simulink model "Synch_Gen1"  (Simulink 4.00)
settings: Solver=ode23tb  StartTime=0.0  StopTime=1
InitFcn:
  | powericon('psbinitsys',bdroot);
libraries: powerlib2 x8, powerlib_extras x3
settings Model: LastModifiedBy=ieao  SaveTime=off  SaveOutput=off  LimitDataPoints=off  BlockReductionOpt=off

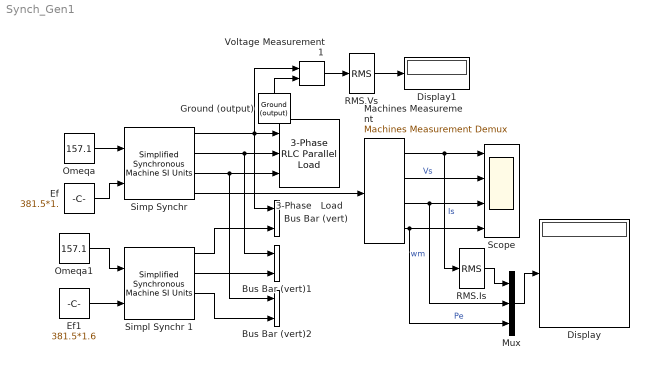
== system Synch_Gen1 ==
  3-Phase   Load : powerlib_extras/Three-Phase Library/3-Phase RLC Parallel Load  Vpp=380  fn=50  P3=100e3  QL3=50e3  QC3=0
  Bus Bar (vert) : powerlib2/Connectors/Bus Bar (vert)  Tag=PoWeRsYsTeMbLoCk  entrees=2  sorties=0  PSBOutputType=11111111111111111111111111111111111111111111111111111111111111111111111111111111111111111
  Bus Bar (vert)1 : powerlib2/Connectors/Bus Bar (vert)  Tag=PoWeRsYsTeMbLoCk  entrees=2  sorties=0  PSBOutputType=11111111111111111111111111111111111111111111111111111111111111111111111111111111111111111
  Bus Bar (vert)2 : powerlib2/Connectors/Bus Bar (vert)  Tag=PoWeRsYsTeMbLoCk  entrees=2  sorties=0  PSBOutputType=11111111111111111111111111111111111111111111111111111111111111111111111111111111111111111
  Display : Display
      settings: Format=short  SampleTime=0
  Display1 : Display
      settings: Format=short  SampleTime=0
  Ef : Constant  Value=381.5*1.
  Ef1 : Constant  Value=381.5*1.6
  Ground (output) : powerlib2/Connectors/Ground (output)  Tag=PoWeRsYsTeMbLoCk  Orientation=up  PSBOutputType=1
  Machines Measurement : powerlib2/Machines/Machines Measurement Demux  machType=Simplified synchronous  ssm1=on  ssm2=on  ssm3=off  ssm4=off  ssm5=on  ssm6=on  sm1=on  sm2=off  sm3=on  sm4=off  sm5=off  sm6=off  sm7=off  sm8=on  sm9=on  sm10=off  sm11=off  asm1=on  asm2=on  asm3=on  asm4=on  asm5=on  asm6=on  asm7=on  asm8=on  asm9=on  asm10=on  asm11=on  pmsm1=on  pmsm2=on  pmsm3=on  pmsm4=on  pmsm5=on  pmsm6=on  lastType=1
  Mux : Mux  Inputs=3
  Omeqa : Constant  Value=157.1
  Omeqa1 : Constant  Value=157.1
  RMS.Is : powerlib_extras/Measurements/RMS  f1=50
  RMS.Vs : powerlib_extras/Measurements/RMS  f1=50
  Scope : Scope  NumInputPorts=4
      settings: TimeRange=auto  YMin=-5~-5~-5~-5  YMax=5~5~5~5  SaveToWorkspace=off  SaveName=ScopeData  MaxDataPoints=5000
  "Simp Synchr " : powerlib2/Machines/Simplified Synchronous  Machine SI Units  Tag=PoWeRsYsTeMbLoCk  conType=3-wire Y  x1=[ 100e3,380,50 ]  x2=[ inf,0,2 ]  x3=[ 0. 0.9e-3 ]  x4="[ 0   0   0,0,0   0,0,0 ]"  PSBOutputType=1111  iounits=1
  Simpl Synchr 1 : powerlib2/Machines/Simplified Synchronous  Machine SI Units  Tag=PoWeRsYsTeMbLoCk  conType=3-wire Y  x1=[100e3,380,50 ]  x2=[ inf,0,2 ]  x3=[ 0. 4.9e-3 ]  x4="[ 0   0   0,0,0   0,0,0 ]"  PSBOutputType=1111  iounits=1
  Voltage Measurement1 : powerlib2/Measurements/Voltage Measurement  Tag=PoWeRsYsTeMmEaSuReMeNt  PSBOutputType=0  PSBequivalent=1
  wires:
  "Simp Synchr "/1 -> 3-Phase   Load/1, Voltage Measurement1/1, Bus Bar (vert)/1
  "Simp Synchr "/2 -> 3-Phase   Load/2, Bus Bar (vert)1/1
  "Simp Synchr "/3 -> 3-Phase   Load/3, Bus Bar (vert)2/1
  "Simp Synchr "/4 -> Machines Measurement/1
  Omeqa/1 -> "Simp Synchr "/1
  Ef/1 -> "Simp Synchr "/2
  Machines Measurement/1 -> Scope/1, RMS.Is/1  "Is"
  Voltage Measurement1/1 -> RMS.Vs/1
  RMS.Vs/1 -> Display1/1
  Ground (output)/1 -> Voltage Measurement1/2
  Machines Measurement/2 -> Scope/2  "Vs"
  Machines Measurement/3 -> Scope/3, Mux/2  "wm"
  Machines Measurement/4 -> Scope/4, Mux/3  "Pe"
  RMS.Is/1 -> Mux/1
  Mux/1 -> Display/1
  Simpl Synchr 1/1 -> Bus Bar (vert)/2
  Simpl Synchr 1/2 -> Bus Bar (vert)1/2
  Simpl Synchr 1/3 -> Bus Bar (vert)2/2
  Ef1/1 -> Simpl Synchr 1/2
  Omeqa1/1 -> Simpl Synchr 1/1
